simulink model "test_WaveletTraj"  (Simulink 10.1)
settings: Solver=FixedStepDiscrete  StartTime=0.0  StopTime=7  FixedStep=Ts  RelTol=1e-3
PreLoadFcn:
  | load param
undefined symbols (not defined in the file or in its folder): c_maxsz, DiscIntNeverNeededParam, Dphival_fi, f, interp_gain, interp_uplim, phival_fi, Ts, tval_fi, w
libraries: simulink x11, dspsigops x6, dspswit3 x3, simulink_extras x2, dspsrcs4 x1
settings Model: Creator=Carchesion  LastModifiedBy=upattacini  ParamWorkspaceSource=ReferencedWorkspace
settings SolverCC: ZeroCrossAlgorithm=Non-adaptive
settings DataIOCC: SignalLoggingSaveFormat=ModelDataLogs  SaveOutput=off  SignalLogging=off  SaveTime=off
settings OptimizationCC: DefaultParameterBehavior=Inlined  InlineInvariantSignals=on  ExpressionDepthLimit=2147483647  StateBitsets=on  DataBitsets=on  NoFixptDivByZeroProtection=on  EfficientFloat2IntCast=on  LifeSpan=1  SimCompilerOptimization=on  EfficientTunableParamExpr=on
settings DebuggingCC: SolverPrmCheckMsg=warning  ParameterPrecisionLossMsg=none  FcnCallInpInsideContextMsg=warning  StateNameClashWarn=warning
settings HardwareCC: ProdIntDivRoundTo=Zero  ProdEndianess=BigEndian  ProdWordSize=16  ProdHWDeviceType=Generic->Custom  TargetBitPerInt=16  TargetIntDivRoundTo=Zero  TargetEndianess=BigEndian  TargetWordSize=16  TargetHWDeviceType=Freescale->DSP563xx (16-bit mode)
settings SFSimCC: SimUseLocalCustomCode=on  SimParseCustomCode=off  MATLABDynamicMemAlloc=off  CustomCodeUndefinedFunction=FilterOut
settings RTWCC: Description=Real-Time Workshop Embedded Coder (no auto configuration)  SystemTargetFile=ert.tlc  GenCodeOnly=on  GenerateMakefile=off  TemplateMakefile=ert_default_tmf  GenerateReport=on  RTWUseLocalCustomCode=on  IncludeHyperlinkInReport=on  LaunchReport=on  PortableWordSizes=on  CreateSILPILBlock=SIL  GenerateTraceInfo=on  RTWCompilerOptimization=on
settings CodeAppCC: ForceParamTrailComments=on  IgnoreCustomStorageClasses=off  SimulinkDataObjDesc=on  CustomSymbolStrType=$R$N$M  CustomSymbolStrFcn=$N$M$F  CustomSymbolStrMacro=$N$M  InsertBlockDesc=on  InternalIdentifier=Classic
settings ERTTargetCC: GenerateSampleERTMain=on  IncludeMdlTerminateFcn=off  SuppressErrorStatus=on  PurelyIntegerCode=on  SupportNonFinite=off  SupportComplex=off  InlinedParameterPlacement=NonHierarchical  ERTCustomFileTemplate=example_file_process.tlc  GlobalDataDefinition=InSourceFile  GlobalDataReference=InSourceFile  ConvertIfToSwitch=off  SuppressUnreachableDefaultCases=off
settings ConfigComp: CovExternalEMLEnable=on

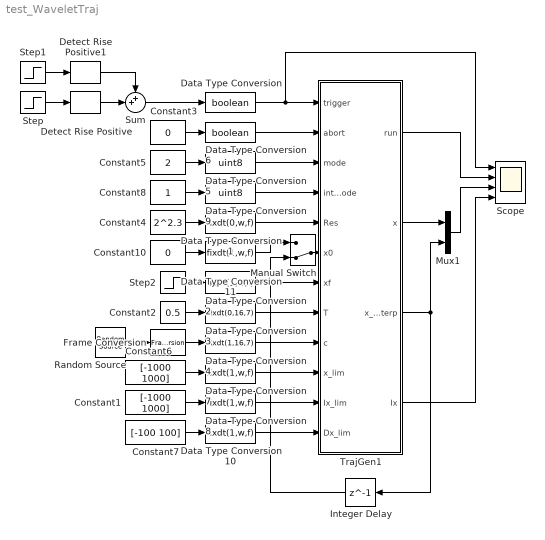
== system test_WaveletTraj ==
  Constant1 : Constant  Value=[-1000 1000]
  Constant10 : Constant  Value=0
  Constant2 : Constant  Value=0.5
  Constant3 : Constant  Value=0
  Constant4 : Constant  Value=2^2.3
  Constant5 : Constant  Value=2
  Constant6 : Constant  Value=[-1000 1000]
  Constant7 : Constant  Value=[-100 100]
  Constant8 : Constant
  Data Type Conversion : DataTypeConversion  OutDataTypeStr=boolean  RndMeth=Nearest  SaturateOnIntegerOverflow=on
  Data Type Conversion1 : DataTypeConversion  OutDataTypeStr=fixdt(0,w,f)  RndMeth=Nearest  SaturateOnIntegerOverflow=on
  Data Type Conversion{2,7..8,10..11} (5 alike) : DataTypeConversion  OutDataTypeStr=fixdt(1,w,f)  RndMeth=Nearest  SaturateOnIntegerOverflow=on
  Data Type Conversion3 : DataTypeConversion  OutDataTypeStr=fixdt(0,16,7)  RndMeth=Nearest  SaturateOnIntegerOverflow=on
  Data Type Conversion4 : DataTypeConversion  OutDataTypeStr=fixdt(1,16,7)  RndMeth=Nearest  SaturateOnIntegerOverflow=on
  Data Type Conversion5 : DataTypeConversion  OutDataTypeStr=uint8  RndMeth=Nearest  SaturateOnIntegerOverflow=on
  Data Type Conversion6 : DataTypeConversion  OutDataTypeStr=boolean  RndMeth=Nearest  SaturateOnIntegerOverflow=on
  Data Type Conversion9 : DataTypeConversion  OutDataTypeStr=uint8  RndMeth=Nearest  SaturateOnIntegerOverflow=on
  Detect Rise Positive : simulink/Logic and Bit Operations/Detect Rise Positive  vinit=0  OutDataTypeStr=uint8
  Detect Rise Positive1 : simulink/Logic and Bit Operations/Detect Rise Positive  vinit=0  OutDataTypeStr=uint8
  Frame Conversion : FrameConversion  OutFrame=Sample-based
  Integer Delay : Delay  DelayLength=1
  Manual Switch : ManualSwitch  CurrentSetting=0
  Mux1 : Mux  Inputs=2
  Random Source : dspsrcs4/Random Source  SrcType=Uniform  NormMethod=Ziggurat  CltLength=12  MinVal=-10  MaxVal=10  MeanVal=0  VarVal=1  RepMode=Not repeatable  rawSeed=1  IsInherit=off  SampMode=Discrete  SampTime=Ts/c_maxsz  SampFrame=c_maxsz  DataType=Double  OutComplex=Real  OutputFrames=on
  Scope : Scope  NumInputPorts=4
  Step : Step  SampleTime=Ts
  Step1 : Step  Time=2  SampleTime=Ts
  Step2 : Step  Time=1.5  Before=10  After=20  SampleTime=Ts
  Sum : Sum  Inputs=++|
  TrajGen1 : Subsystem  TreatAsAtomicUnit=on  RTWFcnName=WaveletTrajectory
      settings: RTWFcnNameOpts=User specified
  wires:
  Constant4/1 -> Data Type Conversion1/1
  Constant2/1 -> Data Type Conversion3/1
  Step/1 -> Detect Rise Positive/1
  Step1/1 -> Detect Rise Positive1/1
  Random Source/1 -> Frame Conversion/1
  Frame Conversion/1 -> Data Type Conversion4/1
  Data Type Conversion/1 -> Scope/1, TrajGen1/1(trigger)
  Sum/1 -> Data Type Conversion/1
  Mux1/1 -> Scope/3
  Data Type Conversion4/1 -> TrajGen1/9(c)
  Data Type Conversion3/1 -> TrajGen1/8(T)
  Data Type Conversion1/1 -> TrajGen1/5(Res)
  Step2/1 -> Data Type Conversion2/1
  Data Type Conversion2/1 -> TrajGen1/7(xf)
  Detect Rise Positive/1 -> Sum/2
  Detect Rise Positive1/1 -> Sum/1
  Data Type Conversion5/1 -> TrajGen1/3(mode)
  Data Type Conversion6/1 -> TrajGen1/2(abort)
  Constant5/1 -> Data Type Conversion5/1
  Data Type Conversion7/1 -> TrajGen1/10(x_lim)
  Data Type Conversion8/1 -> TrajGen1/11(Ix_lim)
  Constant6/1 -> Data Type Conversion7/1
  Constant1/1 -> Data Type Conversion8/1
  Constant3/1 -> Data Type Conversion6/1
  Constant8/1 -> Data Type Conversion9/1
  Data Type Conversion9/1 -> TrajGen1/4(int_mode)
  TrajGen1/1(run) -> Scope/2
  TrajGen1/2(x) -> Mux1/1
  TrajGen1/3(x_interp) -> Mux1/2, Integer Delay/1
  TrajGen1/4(Ix) -> Scope/4
  Data Type Conversion10/1 -> TrajGen1/12(Dx_lim)
  Constant7/1 -> Data Type Conversion10/1
  Manual Switch/1 -> TrajGen1/6(x0)
  Integer Delay/1 -> Manual Switch/2
  Constant10/1 -> Data Type Conversion11/1
  Data Type Conversion11/1 -> Manual Switch/1

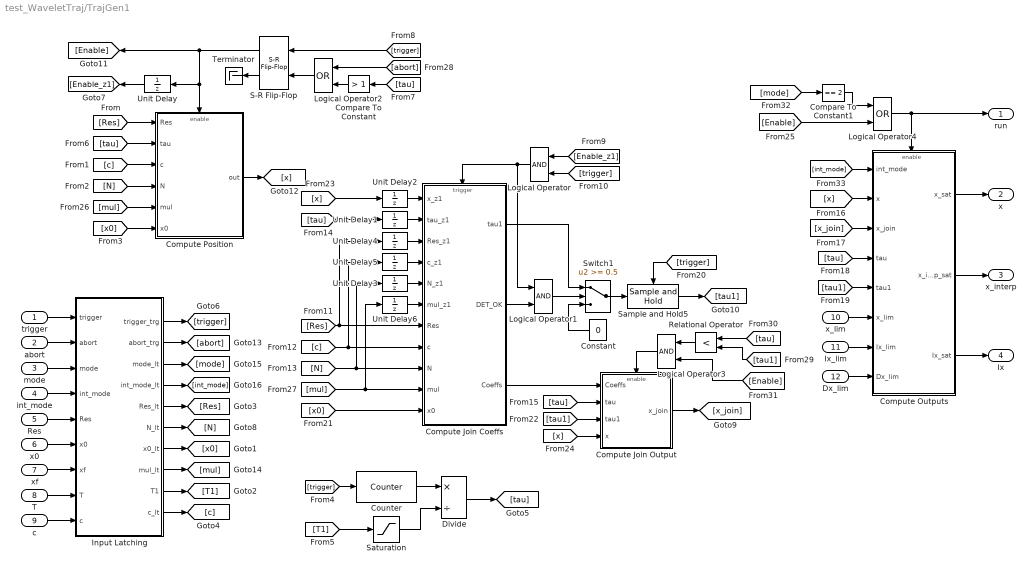
== system test_WaveletTraj/TrajGen1 ==
  trigger : Inport  PortDimensions=1
  abort : Inport  Port=2  PortDimensions=1
  mode : Inport  Port=3  PortDimensions=1
  int_mode : Inport  Port=4  PortDimensions=1
  Res : Inport  Port=5  PortDimensions=1
  x0 : Inport  Port=6  PortDimensions=1
  xf : Inport  Port=7  PortDimensions=1
  T : Inport  Port=8  PortDimensions=1
  c : Inport  Port=9  PortDimensions=c_maxsz
  x_lim : Inport  Port=10  PortDimensions=2
  Ix_lim : Inport  Port=11  PortDimensions=2
  Dx_lim : Inport  Port=12  PortDimensions=2
  Compare To Constant : simulink/Logic and Bit Operations/Compare To Constant  relop=>  const=1  OutDataTypeStr=boolean  ZeroCross=off
  Compare To Constant1 : simulink/Logic and Bit Operations/Compare To Constant  relop===  const=2  OutDataTypeStr=boolean  ZeroCross=off
  Compute Join Coeffs : Subsystem  RTWFcnName=Trajectory_ComputeJoinCoeffs
      settings: RTWFcnNameOpts=User specified
  Compute Join Output : Subsystem  TreatAsAtomicUnit=on  RTWFcnName=Trajectory_ComputeJoinOutput
      settings: RTWFcnNameOpts=User specified
  Compute Outputs : Subsystem  TreatAsAtomicUnit=on  RTWFcnName=Trajectory_ComputeOutputs
      settings: RTWFcnNameOpts=User specified
  Compute Position : Subsystem  TreatAsAtomicUnit=on  RTWFcnName=Trajectory_ComputePosition
      settings: RTWFcnNameOpts=User specified
  Constant : Constant  Value=0  OutDataTypeStr=fixdt(1,w,f)
  Counter : dspswit3/Counter  Direction=Up  CountEvent=Free running  CounterSize=32 bits  MaxCount=255  InitialCount=0  Output=Count  HitValue=32  ResetInput=on  SamplesPerFrame=1  Ts=-1  CntDtype=uint32  HitDtype=Logical
  Divide : Product  Inputs=*/  OutDataTypeStr=fixdt(1,w,f)  RndMeth=Nearest  SaturateOnIntegerOverflow=on
  Input Latching : Subsystem  TreatAsAtomicUnit=on  RTWFcnName=Trajectory_InputLatching
      settings: RTWFcnNameOpts=User specified
  Logical Operator : Logic  IconShape=distinctive  AllPortsSameDT=off  OutDataTypeStr=boolean
  Logical Operator1 : Logic  IconShape=distinctive  AllPortsSameDT=off  OutDataTypeStr=boolean
  Logical Operator2 : Logic  Operator=OR  IconShape=distinctive  AllPortsSameDT=off  OutDataTypeStr=boolean
  Logical Operator3 : Logic  IconShape=distinctive  AllPortsSameDT=off  OutDataTypeStr=boolean
  Logical Operator4 : Logic  Operator=OR  IconShape=distinctive  AllPortsSameDT=off  OutDataTypeStr=boolean
  Relational Operator : RelationalOperator  Operator=<  OutDataTypeStr=boolean  RndMeth=Nearest
  S-R Flip-Flop : simulink_extras/Flip Flops/S-R Flip-Flop  initial_condition=0
  Sample and Hold5 : dspsigops/Sample and Hold  trig=Rising edge  initCond=0  latchinput=off
  Saturation : Saturate  UpperLimit=intmax('uint32')  LowerLimit=1  OutDataTypeStr=uint32  RndMeth=Nearest
  Switch1 : Switch  Threshold=0.5  OutDataTypeStr=fixdt(0,w,f)  RndMeth=Nearest  SaturateOnIntegerOverflow=on
  Terminator : Terminator
  Unit Delay{,1..6} (7 alike) : UnitDelay  SampleTime=-1
  run : Outport  PortDimensions=1
  x : Outport  Port=2  PortDimensions=1
  x_interp : Outport  Port=3  PortDimensions=1
  Ix : Outport  Port=4  PortDimensions=1
  wires:
  Unit Delay4/1 -> Compute Join Coeffs/3(Res_z1)
  [x] -> Compute Join Output/4(x)
  [tau1] -> Compute Join Output/3(tau1)
  Compute Join Output/1(x_join) -> [x_join]
  Unit Delay2/1 -> Compute Join Coeffs/1(x_z1)
  Unit Delay1/1 -> Compute Join Coeffs/2(tau_z1)
  [x0] -> Compute Position/6(x0)
  [x] -> Unit Delay2/1
  [tau] -> Unit Delay1/1
  Logical Operator1/1 -> Switch1/2
  Compute Join Coeffs/2(DET_OK) -> Logical Operator1/2
  [x0] -> Compute Join Coeffs/11(x0)
  [tau] -> Compute Join Output/2(tau)
  Compute Join Coeffs/3(Coeffs) -> Compute Join Output/1(Coeffs)
  [trigger] -> Sample and Hold5/Trigger
  Sample and Hold5/1 -> [tau1]
  Constant/1 -> Switch1/3
  Compute Join Coeffs/1(tau1) -> Switch1/1
  Switch1/1 -> Sample and Hold5/1
  Logical Operator/1 -> Logical Operator1/1, Compute Join Coeffs/Trigger
  [N] -> Compute Join Coeffs/9(N), Unit Delay3/1
  [c] -> Compute Join Coeffs/8(c), Unit Delay5/1
  [Res] -> Unit Delay4/1, Compute Join Coeffs/7(Res)
  Compute Position/1(out) -> [x]
  [trigger] -> Logical Operator/2
  [Enable_z1] -> Logical Operator/1
  [trigger] -> Counter/1
  Counter/1 -> Divide/1
  S-R Flip-Flop/1 -> Compute Position/Enable, Unit Delay/1, [Enable]
  S-R Flip-Flop/2 -> Terminator/1
  [tau] -> Compare To Constant/1
  [trigger] -> S-R Flip-Flop/1
  Saturation/1 -> Divide/2
  [tau] -> Compute Position/2(tau)
  Divide/1 -> [tau]
  [T1] -> Saturation/1
  [N] -> Compute Position/4(N)
  [c] -> Compute Position/3(c)
  [Res] -> Compute Position/1(Res)
  Unit Delay5/1 -> Compute Join Coeffs/4(c_z1)
  Unit Delay3/1 -> Compute Join Coeffs/5(N_z1)
  Unit Delay/1 -> [Enable_z1]
  trigger/1 -> Input Latching/1(trigger)
  mode/1 -> Input Latching/3(mode)
  Res/1 -> Input Latching/5(Res)
  x0/1 -> Input Latching/6(x0)
  T/1 -> Input Latching/8(T)
  c/1 -> Input Latching/9(c)
  xf/1 -> Input Latching/7(xf)
  Input Latching/1(trigger_trg) -> [trigger]
  Input Latching/5(Res_lt) -> [Res]
  Input Latching/6(N_lt) -> [N]
  Input Latching/7(x0_lt) -> [x0]
  Input Latching/9(T1) -> [T1]
  Input Latching/10(c_lt) -> [c]
  Input Latching/8(mul_lt) -> [mul]
  [mul] -> Compute Position/5(mul)
  [mul] -> Compute Join Coeffs/10(mul), Unit Delay6/1
  Unit Delay6/1 -> Compute Join Coeffs/6(mul_z1)
  abort/1 -> Input Latching/2(abort)
  Input Latching/2(abort_trg) -> [abort]
  Logical Operator2/1 -> S-R Flip-Flop/2
  [abort] -> Logical Operator2/1
  x_lim/1 -> Compute Outputs/6(x_lim)
  Ix_lim/1 -> Compute Outputs/7(Ix_lim)
  [tau1] -> Compute Outputs/5(tau1)
  [tau] -> Compute Outputs/4(tau)
  [x_join] -> Compute Outputs/3(x_join)
  [x] -> Compute Outputs/2(x)
  Compute Outputs/1(x_sat) -> x/1
  Compute Outputs/2(x_interp_sat) -> x_interp/1
  Compute Outputs/3(Ix_sat) -> Ix/1
  [tau] -> Relational Operator/1
  [tau1] -> Relational Operator/2
  Relational Operator/1 -> Logical Operator3/1
  Logical Operator3/1 -> Compute Join Output/Enable
  [Enable] -> Logical Operator3/2
  Dx_lim/1 -> Compute Outputs/8(Dx_lim)
  int_mode/1 -> Input Latching/4(int_mode)
  Input Latching/3(mode_lt) -> [mode]
  Input Latching/4(int_mode_lt) -> [int_mode]
  [int_mode] -> Compute Outputs/1(int_mode)
  [mode] -> Compare To Constant1/1
  Compare To Constant/1 -> Logical Operator2/2
  [Enable] -> Logical Operator4/2
  Logical Operator4/1 -> Compute Outputs/Enable, run/1
  Compare To Constant1/1 -> Logical Operator4/1

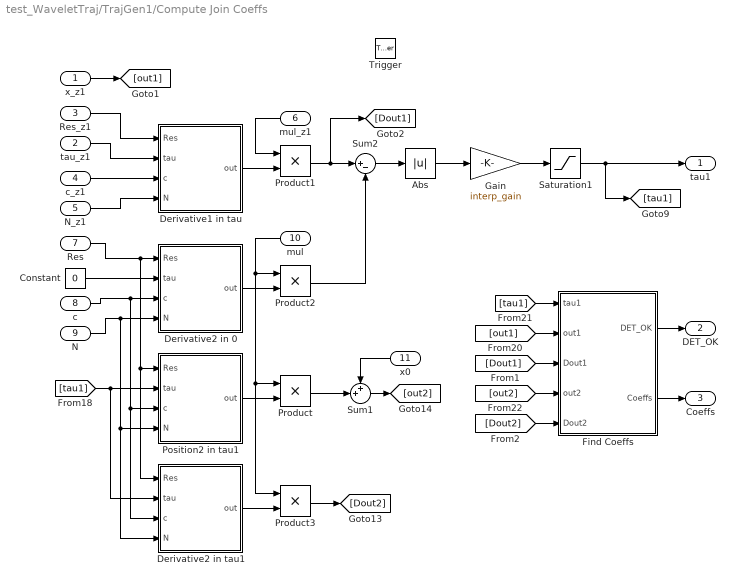
== system test_WaveletTraj/TrajGen1/Compute Join Coeffs ==
  x_z1 : Inport
  tau_z1 : Inport  Port=2
  Res_z1 : Inport  Port=3
  c_z1 : Inport  Port=4
  N_z1 : Inport  Port=5
  mul_z1 : Inport  Port=6
  Res : Inport  Port=7
  c : Inport  Port=8
  N : Inport  Port=9
  mul : Inport  Port=10
  x0 : Inport  Port=11
  Trigger : TriggerPort  VariantControl=(inherit)  StatesWhenEnabling=reset
  Abs : Abs  RndMeth=Nearest  SaturateOnIntegerOverflow=on
  Constant : Constant  Value=0  OutDataTypeStr=fixdt(1,w,f)
  Derivative1 in tau : Subsystem  TreatAsAtomicUnit=on  RTWFcnName=Trajectory_Derivative
      settings: RTWFcnNameOpts=User specified
  Derivative2 in 0 : Subsystem  TreatAsAtomicUnit=on  RTWFcnName=Trajectory_Derivative
      settings: RTWFcnNameOpts=User specified
  Derivative2 in tau1 : Subsystem  TreatAsAtomicUnit=on  RTWFcnName=Trajectory_Derivative
      settings: RTWFcnNameOpts=User specified
  Find Coeffs : Subsystem  TreatAsAtomicUnit=on  RTWFcnName=Trajectory_FindCoeffs
      settings: RTWFcnNameOpts=User specified
  Gain : Gain  Gain=interp_gain  ParamDataTypeStr=fixdt(1,w,f)  RndMeth=Nearest  SaturateOnIntegerOverflow=on  OutDataTypeStr=Inherit: Same as input
  Position2 in tau1 : Subsystem  TreatAsAtomicUnit=on  RTWFcnName=Trajectory_Position
      settings: RTWFcnNameOpts=User specified
  Product{,1..3} (4 alike) : Product  OutDataTypeStr=fixdt(1,w,f)  RndMeth=Nearest  SaturateOnIntegerOverflow=on
  Saturation1 : Saturate  UpperLimit=interp_uplim  LowerLimit=0  OutDataTypeStr=fixdt(1,w,f)  RndMeth=Nearest
  Sum1 : Sum  Inputs=++|  OutDataTypeStr=fixdt(1,w,f)  RndMeth=Nearest  SaturateOnIntegerOverflow=on
  Sum2 : Sum  Inputs=|+-  OutDataTypeStr=fixdt(1,w,f)  RndMeth=Nearest  SaturateOnIntegerOverflow=on
  tau1 : Outport
  DET_OK : Outport  Port=2
  Coeffs : Outport  Port=3
  wires:
  N_z1/1 -> Derivative1 in tau/4(N)
  Res_z1/1 -> Derivative1 in tau/1(Res)
  Find Coeffs/1(DET_OK) -> DET_OK/1
  tau_z1/1 -> Derivative1 in tau/2(tau)
  c_z1/1 -> Derivative1 in tau/3(c)
  x0/1 -> Sum1/1
  Sum1/1 -> [out2]
  Saturation1/1 -> [tau1], tau1/1
  Find Coeffs/2(Coeffs) -> Coeffs/1
  [Dout2] -> Find Coeffs/5(Dout2)
  [out2] -> Find Coeffs/4(out2)
  [Dout1] -> Find Coeffs/3(Dout1)
  [out1] -> Find Coeffs/2(out1)
  [tau1] -> Find Coeffs/1(tau1)
  x_z1/1 -> [out1]
  [tau1] -> Derivative2 in tau1/2(tau), Position2 in tau1/2(tau)
  Gain/1 -> Saturation1/1
  Abs/1 -> Gain/1
  Sum2/1 -> Abs/1
  N/1 -> Derivative2 in 0/4(N), Derivative2 in tau1/4(N), Position2 in tau1/4(N)
  c/1 -> Derivative2 in 0/3(c), Derivative2 in tau1/3(c), Position2 in tau1/3(c)
  Constant/1 -> Derivative2 in 0/2(tau)
  Res/1 -> Derivative2 in 0/1(Res), Derivative2 in tau1/1(Res), Position2 in tau1/1(Res)
  Product/1 -> Sum1/2
  Derivative1 in tau/1(out) -> Product1/2
  Product1/1 -> Sum2/1, [Dout1]
  mul_z1/1 -> Product1/1
  Derivative2 in 0/1(out) -> Product2/2
  Product2/1 -> Sum2/2
  Derivative2 in tau1/1(out) -> Product3/2
  Product3/1 -> [Dout2]
  Position2 in tau1/1(out) -> Product/2
  mul/1 -> Product2/1, Product/1, Product3/1

== system test_WaveletTraj/TrajGen1/Compute Join Output ==
  Coeffs : Inport
  tau : Inport  Port=2
  tau1 : Inport  Port=3
  x : Inport  Port=4
  Enable : EnablePort
  CalcPoly : Subsystem
  CalcRho : Subsystem
  Product : Product  OutDataTypeStr=fixdt(1,w,f)  RndMeth=Nearest  SaturateOnIntegerOverflow=on
  Product1 : Product  OutDataTypeStr=fixdt(1,w,f)  RndMeth=Nearest  SaturateOnIntegerOverflow=on
  Sum2 : Sum  Inputs=|++  OutDataTypeStr=fixdt(1,w,f)  RndMeth=Nearest  SaturateOnIntegerOverflow=on
  x_join : Outport
  wires:
  x/1 -> Product1/2
  CalcRho/2(Rho2) -> Product1/1
  Sum2/1 -> x_join/1
  Product1/1 -> Sum2/2
  Product/1 -> Sum2/1
  CalcRho/1(Rho1) -> Product/2
  CalcPoly/1(out_poly3) -> Product/1
  tau1/1 -> CalcRho/2(tau1)
  Coeffs/1 -> CalcPoly/2(Coeffs)
  tau/1 -> CalcRho/1(tau), CalcPoly/1(tau)

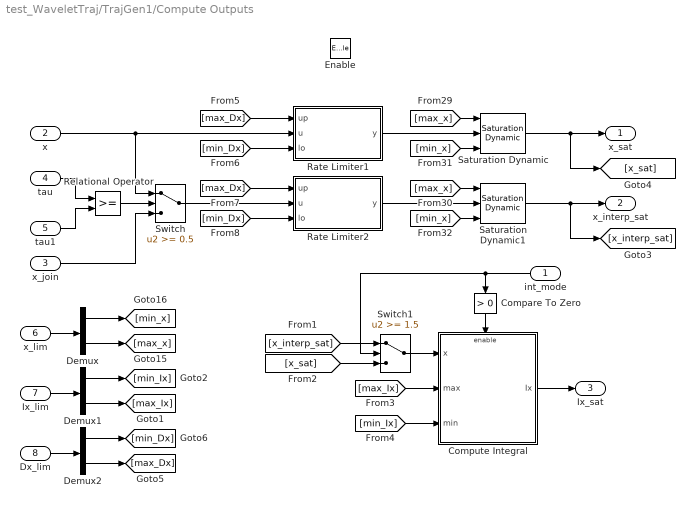
== system test_WaveletTraj/TrajGen1/Compute Outputs ==
  int_mode : Inport
  x : Inport  Port=2
  x_join : Inport  Port=3
  tau : Inport  Port=4
  tau1 : Inport  Port=5
  x_lim : Inport  Port=6
  Ix_lim : Inport  Port=7
  Dx_lim : Inport  Port=8
  Enable : EnablePort
  Compare To Zero : simulink/Logic and Bit Operations/Compare To Zero  relop=>  OutDataTypeStr=boolean  ZeroCross=off
  Compute Integral : Subsystem  TreatAsAtomicUnit=on  RTWFcnName=Trajectory_ComputeIntegral
      settings: RTWFcnNameOpts=User specified
  Demux : Demux  Outputs=2
  Demux1 : Demux  Outputs=2
  Demux2 : Demux  Outputs=2
  Rate Limiter1 : Subsystem  TreatAsAtomicUnit=on  RTWFcnName=Trajectory_RateLimiter
      settings: RTWFcnNameOpts=User specified
      mask Display:
      | disp('Rate\nLimiter');
      | port_label('input',1,'up');
      | port_label('input',2,'u');
      | port_label('input',3,'lo');
      | port_label('output',1,'y');
  Rate Limiter2 : Subsystem  TreatAsAtomicUnit=on  RTWFcnName=Trajectory_RateLimiter
      settings: RTWFcnNameOpts=User specified
      mask Display:
      | disp('Rate\nLimiter');
      | port_label('input',1,'up');
      | port_label('input',2,'u');
      | port_label('input',3,'lo');
      | port_label('output',1,'y');
  Relational Operator : RelationalOperator  OutDataTypeStr=boolean  RndMeth=Nearest
  Saturation Dynamic : simulink/Discontinuities/Saturation Dynamic  OutMin=[]  OutMax=[]  OutDataTypeStr=fixdt(1,w,f)  OutputDataTypeScalingMode=Specify via dialog  OutDataType=fixdt(1,w,f)  OutScaling=[]  RndMeth=Nearest  DoSatur=on
  Saturation Dynamic1 : simulink/Discontinuities/Saturation Dynamic  OutMin=[]  OutMax=[]  OutDataTypeStr=fixdt(1,w,f)  OutputDataTypeScalingMode=Specify via dialog  OutDataType=fixdt(1,w,f)  OutScaling=[]  RndMeth=Nearest  DoSatur=on
  Switch : Switch  Threshold=0.5  OutDataTypeStr=fixdt(1,w,f)  RndMeth=Nearest  SaturateOnIntegerOverflow=on
  Switch1 : Switch  Threshold=1.5  OutDataTypeStr=fixdt(1,w,f)  RndMeth=Nearest  SaturateOnIntegerOverflow=on
  x_sat : Outport
  x_interp_sat : Outport  Port=2
  Ix_sat : Outport  Port=3
  wires:
  x/1 -> Switch/1, Rate Limiter1/2(u)
  [min_x] -> Saturation Dynamic1/3
  [min_x] -> Saturation Dynamic/3
  [max_x] -> Saturation Dynamic1/1
  [max_x] -> Saturation Dynamic/1
  Relational Operator/1 -> Switch/2
  Saturation Dynamic/1 -> x_sat/1, [x_sat]
  tau/1 -> Relational Operator/1
  Saturation Dynamic1/1 -> x_interp_sat/1, [x_interp_sat]
  tau1/1 -> Relational Operator/2
  x_join/1 -> Switch/3
  Demux/1 -> [min_x]
  Demux/2 -> [max_x]
  Demux1/1 -> [min_Ix]
  Demux1/2 -> [max_Ix]
  [max_Ix] -> Compute Integral/2(max)
  [min_Ix] -> Compute Integral/3(min)
  Compute Integral/1(Ix) -> Ix_sat/1
  x_lim/1 -> Demux/1
  Ix_lim/1 -> Demux1/1
  [x_interp_sat] -> Switch1/1
  [x_sat] -> Switch1/3
  Switch1/1 -> Compute Integral/1(x)
  int_mode/1 -> Compare To Zero/1, Switch1/2
  Compare To Zero/1 -> Compute Integral/Enable
  Demux2/1 -> [min_Dx]
  Demux2/2 -> [max_Dx]
  Dx_lim/1 -> Demux2/1
  Rate Limiter1/1(y) -> Saturation Dynamic/2
  Rate Limiter2/1(y) -> Saturation Dynamic1/2
  Switch/1 -> Rate Limiter2/2(u)
  [max_Dx] -> Rate Limiter1/1(up)
  [min_Dx] -> Rate Limiter1/3(lo)
  [min_Dx] -> Rate Limiter2/3(lo)
  [max_Dx] -> Rate Limiter2/1(up)

== system test_WaveletTraj/TrajGen1/Compute Position ==
  Res : Inport  PortDimensions=1
  tau : Inport  Port=2  PortDimensions=1
  c : Inport  Port=3  PortDimensions=c_maxsz
  N : Inport  Port=4  PortDimensions=1
  mul : Inport  Port=5  PortDimensions=1
  x0 : Inport  Port=6  PortDimensions=1
  Enable : EnablePort
  Position : Subsystem  TreatAsAtomicUnit=on  RTWFcnName=Trajectory_Position
      settings: RTWFcnNameOpts=User specified
  Product : Product  OutDataTypeStr=fixdt(1,w,f)  RndMeth=Nearest  SaturateOnIntegerOverflow=on
  Sum1 : Sum  Inputs=|++  OutDataTypeStr=fixdt(1,w,f)  RndMeth=Nearest  SaturateOnIntegerOverflow=on
  out : Outport  PortDimensions=1
  wires:
  x0/1 -> Sum1/2
  Sum1/1 -> out/1
  N/1 -> Position/4(N)
  c/1 -> Position/3(c)
  tau/1 -> Position/2(tau)
  Res/1 -> Position/1(Res)
  Position/1(out) -> Product/1
  Product/1 -> Sum1/1
  mul/1 -> Product/2

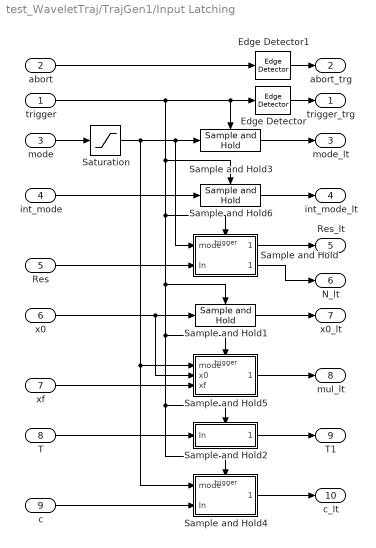
== system test_WaveletTraj/TrajGen1/Input Latching ==
  trigger : Inport
  abort : Inport  Port=2
  mode : Inport  Port=3
  int_mode : Inport  Port=4
  Res : Inport  Port=5
  x0 : Inport  Port=6
  xf : Inport  Port=7
  T : Inport  Port=8
  c : Inport  Port=9
  Edge Detector : dspswit3/Edge Detector  InputProcessing=Columns as channels (frame based)
      settings: SourceProductBaseCode=DS
  Edge Detector1 : dspswit3/Edge Detector  InputProcessing=Columns as channels (frame based)
      settings: SourceProductBaseCode=DS
  Sample and Hold : Subsystem  TreatAsAtomicUnit=on  mask(Sample and Hold){trig=Rising edge, initCond=0, latchinput=off}
      mask prompts: trig "Trigger type:"; initCond "Initial condition:"; latchinput "Latch (buffer) input"
      mask help: Sample and hold the input signal. If Latch (buffer) input is selected, then this block produces the value of the input from the previous time step.
      mask init:
      | switch trig
      | case 1, s='rising';
      | case 2, s='falling';
      | case 3, s='either';
      | end
      | set_param([gcb '/Trigger'],'triggertype',s);
      | if (latchinput == 1)
      | 	set_param([gcb '/In'],'latchinput','on');
      | 	set_param([gcb '/mode'],'latchinput','on');
      | else
      | 	set_param([gcb '/In'],'latchinput','off');
      | 	set_param([gcb '/mode'],'latchinput','off');
      | end
      mask Help: eval('blocksethelp');
      mask TypeOptions trig: Rising edge | Falling edge | Either edge
      mask Display: disp('S/H')
  Sample and Hold1 : dspsigops/Sample and Hold  trig=Rising edge  initCond=0  latchinput=off
  Sample and Hold2 : Subsystem  TreatAsAtomicUnit=on  mask(Sample and Hold){trig=Rising edge, initCond=0, latchinput=off}
      mask prompts: trig "Trigger type:"; initCond "Initial condition:"; latchinput "Latch (buffer) input"
      mask help: Sample and hold the input signal. If Latch (buffer) input is selected, then this block produces the value of the input from the previous time step.
      mask init:
      | switch trig
      | case 1, s='rising';
      | case 2, s='falling';
      | case 3, s='either';
      | end
      | set_param([gcb '/Trigger'],'triggertype',s);
      | if (latchinput == 1)
      | 	set_param([gcb '/In'],'latchinput','on');
      | else
      | 	set_param([gcb '/In'],'latchinput','off');
      | end
      mask Help: eval('blocksethelp');
      mask TypeOptions trig: Rising edge | Falling edge | Either edge
      mask Display: disp('S/H')
  Sample and Hold3 : dspsigops/Sample and Hold  trig=Rising edge  initCond=0  latchinput=off
  Sample and Hold4 : Subsystem  TreatAsAtomicUnit=on  mask(Sample and Hold){trig=Rising edge, initCond=0, latchinput=off}
      mask prompts: trig "Trigger type:"; initCond "Initial condition:"; latchinput "Latch (buffer) input"
      mask help: Sample and hold the input signal. If Latch (buffer) input is selected, then this block produces the value of the input from the previous time step.
      mask init: same as test_WaveletTraj/TrajGen1/Input Latching/Sample and Hold
      mask Help: eval('blocksethelp');
      mask TypeOptions trig: Rising edge | Falling edge | Either edge
      mask Display: disp('S/H')
  Sample and Hold5 : Subsystem  TreatAsAtomicUnit=on  mask(Sample and Hold){trig=Rising edge, initCond=0, latchinput=off}
      mask prompts: trig "Trigger type:"; initCond "Initial condition:"; latchinput "Latch (buffer) input"
      mask help: Sample and hold the input signal. If Latch (buffer) input is selected, then this block produces the value of the input from the previous time step.
      mask init:
      | switch trig
      | case 1, s='rising';
      | case 2, s='falling';
      | case 3, s='either';
      | end
      | set_param([gcb '/Trigger'],'triggertype',s);
      | if (latchinput == 1)
      | 	set_param([gcb '/mode'],'latchinput','on');
      | 	set_param([gcb '/x0'],'latchinput','on');
      | 	set_param([gcb '/xf'],'latchinput','on');
      | else
      | 	set_param([gcb '/mode'],'latchinput','off');
      | 	set_param([gcb '/x0'],'latchinput','off');
      | 	set_param([gcb '/xf'],'latchinput','off');
      | end
      mask Help: eval('blocksethelp');
      mask TypeOptions trig: Rising edge | Falling edge | Either edge
      mask Display: disp('S/H')
  Sample and Hold6 : dspsigops/Sample and Hold  trig=Rising edge  initCond=0  latchinput=off
  Saturation : Saturate  UpperLimit=2  LowerLimit=0  OutDataTypeStr=uint8  RndMeth=Nearest
  trigger_trg : Outport
  abort_trg : Outport  Port=2
  mode_lt : Outport  Port=3
  int_mode_lt : Outport  Port=4
  Res_lt : Outport  Port=5
  N_lt : Outport  Port=6
  x0_lt : Outport  Port=7
  mul_lt : Outport  Port=8
  T1 : Outport  Port=9
  c_lt : Outport  Port=10
  wires:
  Sample and Hold4/1(" ") -> c_lt/1
  Sample and Hold2/1(" ") -> T1/1
  T/1 -> Sample and Hold2/1(In)
  Sample and Hold1/1 -> x0_lt/1
  x0/1 -> Sample and Hold1/1, Sample and Hold5/2(x0)
  Sample and Hold/2(" 1") -> N_lt/1
  Res/1 -> Sample and Hold/2(In)
  Sample and Hold/1(" ") -> Res_lt/1
  Edge Detector/1 -> trigger_trg/1
  trigger/1 -> Edge Detector/1, Sample and Hold3/Trigger, Sample and Hold1/Trigger, Sample and Hold5/Trigger, Sample and Hold2/Trigger, Sample and Hold4/Trigger, Sample and Hold/Trigger, Sample and Hold6/Trigger
  mode/1 -> Saturation/1
  xf/1 -> Sample and Hold5/3(xf)
  Sample and Hold5/1(" ") -> mul_lt/1
  c/1 -> Sample and Hold4/2(In)
  abort/1 -> Edge Detector1/1
  Edge Detector1/1 -> abort_trg/1
  Sample and Hold3/1 -> mode_lt/1
  Sample and Hold6/1 -> int_mode_lt/1
  int_mode/1 -> Sample and Hold6/1
  Saturation/1 -> Sample and Hold4/1(mode), Sample and Hold5/1(mode), Sample and Hold/1(mode), Sample and Hold3/1

== system test_WaveletTraj/TrajGen1/Compute Join Coeffs/Derivative1 in tau ==
  Res : Inport
  tau : Inport  Port=2
  c : Inport  Port=3
  N : Inport  Port=4
  Derivative : Subsystem  RTWFcnName=Trajectory_Derivative
  out : Outport
  wires:
  N/1 -> Derivative/4(N)
  c/1 -> Derivative/3(c)
  Derivative/1(Dout) -> out/1
  tau/1 -> Derivative/2(tau)
  Res/1 -> Derivative/1(Res)

== system test_WaveletTraj/TrajGen1/Compute Join Coeffs/Derivative2 in 0 ==
  Res : Inport
  tau : Inport  Port=2
  c : Inport  Port=3
  N : Inport  Port=4
  Derivative : Subsystem  RTWFcnName=Trajectory_Derivative
  out : Outport
  wires:
  Res/1 -> Derivative/1(Res)
  tau/1 -> Derivative/2(tau)
  Derivative/1(Dout) -> out/1
  c/1 -> Derivative/3(c)
  N/1 -> Derivative/4(N)

== system test_WaveletTraj/TrajGen1/Compute Join Coeffs/Derivative2 in tau1 ==
  Res : Inport
  tau : Inport  Port=2
  c : Inport  Port=3
  N : Inport  Port=4
  Derivative : Subsystem  RTWFcnName=Trajectory_Derivative
  out : Outport
  wires:
  N/1 -> Derivative/4(N)
  c/1 -> Derivative/3(c)
  Derivative/1(Dout) -> out/1
  tau/1 -> Derivative/2(tau)
  Res/1 -> Derivative/1(Res)

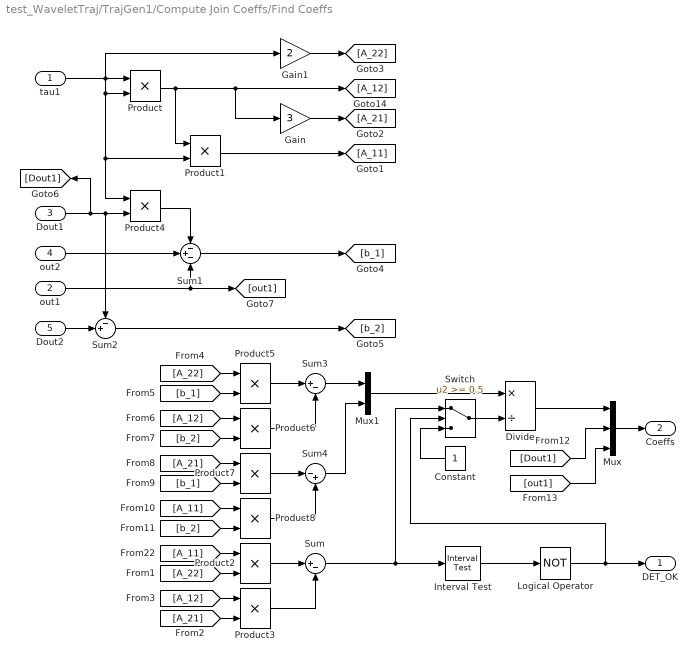
== system test_WaveletTraj/TrajGen1/Compute Join Coeffs/Find Coeffs ==
  tau1 : Inport
  out1 : Inport  Port=2
  Dout1 : Inport  Port=3
  out2 : Inport  Port=4
  Dout2 : Inport  Port=5
  Constant : Constant  OutDataTypeStr=fixdt(1,w,f)
  Divide : Product  Inputs=*/  OutDataTypeStr=fixdt(1,w,f)  RndMeth=Nearest  SaturateOnIntegerOverflow=on
  Gain : Gain  Gain=3  RndMeth=Nearest  SaturateOnIntegerOverflow=on  OutDataTypeStr=Inherit: Same as input  ParamDataTypeStr=Inherit: Same as input
  Gain1 : Gain  Gain=2  RndMeth=Nearest  SaturateOnIntegerOverflow=on  OutDataTypeStr=Inherit: Same as input  ParamDataTypeStr=Inherit: Same as input
  Interval Test : simulink/Logic and Bit Operations/Interval Test  IntervalClosedRight=on  uplimit=2^-f  IntervalClosedLeft=on  lowlimit=-2^-f  OutDataTypeStr=boolean
  Logical Operator : Logic  Operator=NOT  IconShape=distinctive  AllPortsSameDT=off  OutDataTypeStr=boolean
  Mux : Mux  Inputs=3
  Mux1 : Mux  Inputs=2
  Product{,1..8} (9 alike) : Product  OutDataTypeStr=fixdt(1,w,f)  RndMeth=Nearest  SaturateOnIntegerOverflow=on
  Sum : Sum  Inputs=|+-  OutDataTypeStr=fixdt(1,w,f)  RndMeth=Nearest  SaturateOnIntegerOverflow=on
  Sum1 : Sum  Inputs=-+-  OutDataTypeStr=fixdt(1,w,f)  RndMeth=Nearest  SaturateOnIntegerOverflow=on
  Sum2 : Sum  Inputs=-+|  OutDataTypeStr=fixdt(1,w,f)  RndMeth=Nearest  SaturateOnIntegerOverflow=on
  Sum3 : Sum  Inputs=|+-  OutDataTypeStr=fixdt(1,w,f)  RndMeth=Nearest  SaturateOnIntegerOverflow=on
  Sum4 : Sum  Inputs=|-+  OutDataTypeStr=fixdt(1,w,f)  RndMeth=Nearest  SaturateOnIntegerOverflow=on
  Switch : Switch  Threshold=0.5  OutDataTypeStr=fixdt(1,w,f)  RndMeth=Nearest  SaturateOnIntegerOverflow=on
  DET_OK : Outport
  Coeffs : Outport  Port=2
  wires:
  Constant/1 -> Switch/3
  Switch/1 -> Divide/2
  Logical Operator/1 -> Switch/2, DET_OK/1
  Interval Test/1 -> Logical Operator/1
  Mux/1 -> Coeffs/1
  [out1] -> Mux/3
  [Dout1] -> Mux/2
  Divide/1 -> Mux/1
  Sum/1 -> Switch/1, Interval Test/1
  Mux1/1 -> Divide/1
  Sum4/1 -> Mux1/2
  Sum3/1 -> Mux1/1
  Product8/1 -> Sum4/2
  Product7/1 -> Sum4/1
  [b_2] -> Product8/2
  [A_11] -> Product8/1
  [b_1] -> Product7/2
  [A_21] -> Product7/1
  Product6/1 -> Sum3/2
  Product5/1 -> Sum3/1
  [b_2] -> Product6/2
  [A_12] -> Product6/1
  [b_1] -> Product5/2
  [A_22] -> Product5/1
  Sum2/1 -> [b_2]
  Sum1/1 -> [b_1]
  Dout2/1 -> Sum2/2
  Product4/1 -> Sum1/1
  out1/1 -> [out1], Sum1/3
  out2/1 -> Sum1/2
  Dout1/1 -> [Dout1], Sum2/1, Product4/2
  Product3/1 -> Sum/2
  Product2/1 -> Sum/1
  [A_21] -> Product3/2
  [A_12] -> Product3/1
  [A_22] -> Product2/2
  [A_11] -> Product2/1
  Gain1/1 -> [A_22]
  Gain/1 -> [A_21]
  Product1/1 -> [A_11]
  Product/1 -> Gain/1, [A_12], Product1/1
  tau1/1 -> Gain1/1, Product4/1, Product1/2, Product/2, Product/1

== system test_WaveletTraj/TrajGen1/Compute Join Coeffs/Position2 in tau1 ==
  Res : Inport
  tau : Inport  Port=2
  c : Inport  Port=3
  N : Inport  Port=4
  Position : Subsystem  RTWFcnName=Trajectory_Position
  out : Outport
  wires:
  Res/1 -> Position/1(Res)
  tau/1 -> Position/2(tau)
  Position/1(out) -> out/1
  c/1 -> Position/3(c)
  N/1 -> Position/4(N)

== system test_WaveletTraj/TrajGen1/Compute Join Output/CalcPoly ==
  tau : Inport
  Coeffs : Inport  Port=2
  Add : Sum  Inputs=4  OutDataTypeStr=fixdt(1,w,f)  RndMeth=Nearest  SaturateOnIntegerOverflow=on
  Demux : Demux
  Product{,1..4} (5 alike) : Product  OutDataTypeStr=fixdt(1,w,f)  RndMeth=Nearest  SaturateOnIntegerOverflow=on
  out_poly3 : Outport
  wires:
  Coeffs/1 -> Demux/1
  Add/1 -> out_poly3/1
  Demux/4 -> Add/4
  Product4/1 -> Add/3
  Product2/1 -> Add/2
  Product3/1 -> Add/1
  Demux/3 -> Product4/2
  Demux/2 -> Product3/2
  Demux/1 -> Product2/2
  Product1/1 -> Product2/1
  Product/1 -> Product3/1, Product1/1
  tau/1 -> Product4/1, Product1/2, Product/2, Product/1

== system test_WaveletTraj/TrajGen1/Compute Join Output/CalcRho ==
  tau : Inport
  tau1 : Inport  Port=2
  Constant : Constant  OutDataTypeStr=fixdt(1,w,f)
  Divide : Product  Inputs=*/  OutDataTypeStr=fixdt(1,w,f)  RndMeth=Nearest  SaturateOnIntegerOverflow=on
  Product : Product  OutDataTypeStr=fixdt(1,w,f)  RndMeth=Nearest  SaturateOnIntegerOverflow=on
  Saturation1 : Saturate  UpperLimit=2^(w-f-1)  LowerLimit=2^-f  OutDataTypeStr=fixdt(1,w,f)  RndMeth=Nearest
  Sum1 : Sum  Inputs=|+-  OutDataTypeStr=fixdt(1,w,f)  RndMeth=Nearest  SaturateOnIntegerOverflow=on
  Sum2 : Sum  Inputs=-+|  OutDataTypeStr=fixdt(1,w,f)  RndMeth=Nearest  SaturateOnIntegerOverflow=on
  Rho1 : Outport
  Rho2 : Outport  Port=2
  wires:
  Sum2/1 -> Rho2/1
  Saturation1/1 -> Divide/2
  Product/1 -> Sum2/1, Rho1/1
  Sum1/1 -> Product/2, Product/1
  Constant/1 -> Sum2/2, Sum1/2
  Divide/1 -> Sum1/1
  tau1/1 -> Saturation1/1
  tau/1 -> Divide/1

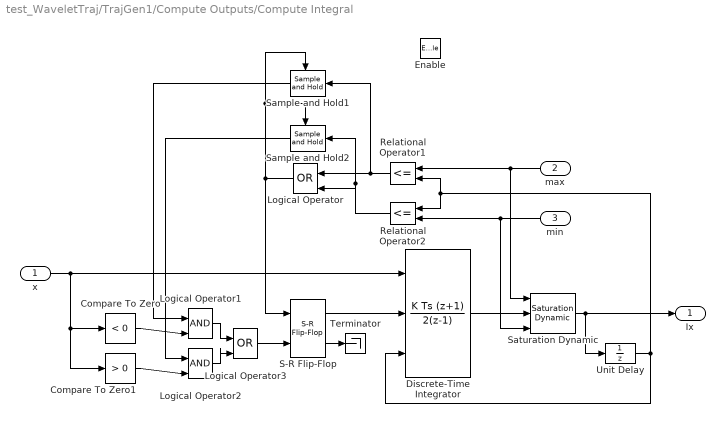
== system test_WaveletTraj/TrajGen1/Compute Outputs/Compute Integral ==
  x : Inport
  max : Inport  Port=2
  min : Inport  Port=3
  Enable : EnablePort
  Compare To Zero : simulink/Logic and Bit Operations/Compare To Zero  relop=<  OutDataTypeStr=boolean  ZeroCross=off
  Compare To Zero1 : simulink/Logic and Bit Operations/Compare To Zero  relop=>  OutDataTypeStr=boolean  ZeroCross=off
  Discrete-Time Integrator : DiscreteIntegrator  IntegratorMethod=Integration: Trapezoidal  ExternalReset=level  InitialConditionSource=external  SampleTime=Ts  OutDataTypeStr=fixdt(1,w,f)  RndMeth=Nearest  SaturateOnIntegerOverflow=on  ICPrevOutput=DiscIntNeverNeededParam  ICPrevScaledInput=DiscIntNeverNeededParam
  Logical Operator : Logic  Operator=OR  IconShape=distinctive  AllPortsSameDT=off  OutDataTypeStr=boolean
  Logical Operator1 : Logic  IconShape=distinctive  AllPortsSameDT=off  OutDataTypeStr=boolean
  Logical Operator2 : Logic  IconShape=distinctive  AllPortsSameDT=off  OutDataTypeStr=boolean
  Logical Operator3 : Logic  Operator=OR  IconShape=distinctive  AllPortsSameDT=off  OutDataTypeStr=boolean
  Relational Operator1 : RelationalOperator  Operator=<=  OutDataTypeStr=boolean  RndMeth=Nearest
  Relational Operator2 : RelationalOperator  Operator=<=  OutDataTypeStr=boolean  RndMeth=Nearest
  S-R Flip-Flop : simulink_extras/Flip Flops/S-R Flip-Flop  initial_condition=0
  Sample and Hold1 : dspsigops/Sample and Hold  trig=Either edge  initCond=0  latchinput=off
  Sample and Hold2 : dspsigops/Sample and Hold  trig=Either edge  initCond=0  latchinput=off
  Saturation Dynamic : simulink/Discontinuities/Saturation Dynamic  OutMin=[]  OutMax=[]  OutDataTypeStr=fixdt(1,w,f)  OutputDataTypeScalingMode=Specify via dialog  OutDataType=fixdt(1,w,f)  OutScaling=[]  RndMeth=Nearest  DoSatur=on
  Terminator : Terminator
  Unit Delay : UnitDelay  SampleTime=-1
  Ix : Outport
  wires:
  max/1 -> Relational Operator1/1, Saturation Dynamic/1
  min/1 -> Relational Operator2/2, Saturation Dynamic/3
  Relational Operator1/1 -> Logical Operator/1, Sample and Hold1/1
  Relational Operator2/1 -> Sample and Hold2/1, Logical Operator/2
  Discrete-Time Integrator/1 -> Saturation Dynamic/2
  Saturation Dynamic/1 -> Ix/1, Unit Delay/1
  x/1 -> Discrete-Time Integrator/1, Compare To Zero/1, Compare To Zero1/1
  Unit Delay/1 -> Discrete-Time Integrator/3, Relational Operator1/2, Relational Operator2/1
  S-R Flip-Flop/1 -> Discrete-Time Integrator/2
  S-R Flip-Flop/2 -> Terminator/1
  Logical Operator/1 -> S-R Flip-Flop/1, Sample and Hold1/Trigger, Sample and Hold2/Trigger
  Compare To Zero/1 -> Logical Operator1/2
  Compare To Zero1/1 -> Logical Operator2/2
  Logical Operator1/1 -> Logical Operator3/1
  Logical Operator2/1 -> Logical Operator3/2
  Logical Operator3/1 -> S-R Flip-Flop/2
  Sample and Hold1/1 -> Logical Operator1/1
  Sample and Hold2/1 -> Logical Operator2/1

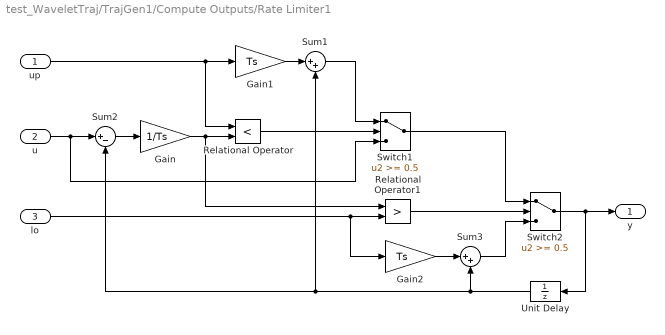
== system test_WaveletTraj/TrajGen1/Compute Outputs/Rate Limiter1 ==
  up : Inport
  u : Inport  Port=2
  lo : Inport  Port=3
  Gain : Gain  Gain=1/Ts  ParamDataTypeStr=fixdt(1,w,f)  RndMeth=Nearest  SaturateOnIntegerOverflow=on  OutDataTypeStr=Inherit: Same as input
  Gain1 : Gain  Gain=Ts  ParamDataTypeStr=fixdt(1,w,f)  OutDataTypeStr=fixdt(1,w,f)  RndMeth=Nearest  SaturateOnIntegerOverflow=on
  Gain2 : Gain  Gain=Ts  ParamDataTypeStr=fixdt(1,w,f)  OutDataTypeStr=fixdt(1,w,f)  RndMeth=Nearest  SaturateOnIntegerOverflow=on
  Relational Operator : RelationalOperator  Operator=<  OutDataTypeStr=boolean  RndMeth=Nearest
  Relational Operator1 : RelationalOperator  Operator=>  OutDataTypeStr=boolean  RndMeth=Nearest
  Sum1 : Sum  Inputs=|++  OutDataTypeStr=fixdt(1,w,f)  RndMeth=Nearest  SaturateOnIntegerOverflow=on
  Sum2 : Sum  Inputs=|+-  OutDataTypeStr=fixdt(1,w,f)  RndMeth=Nearest  SaturateOnIntegerOverflow=on
  Sum3 : Sum  Inputs=|++  OutDataTypeStr=fixdt(1,w,f)  RndMeth=Nearest  SaturateOnIntegerOverflow=on
  Switch1 : Switch  Threshold=0.5  OutDataTypeStr=fixdt(1,w,f)  RndMeth=Nearest  SaturateOnIntegerOverflow=on
  Switch2 : Switch  Threshold=0.5  OutDataTypeStr=fixdt(1,w,f)  RndMeth=Nearest  SaturateOnIntegerOverflow=on
  Unit Delay : UnitDelay  SampleTime=-1
  y : Outport
  wires:
  u/1 -> Sum2/1, Switch1/3
  Sum2/1 -> Gain/1
  Unit Delay/1 -> Sum2/2, Sum1/2, Sum3/2
  Gain/1 -> Relational Operator/2, Relational Operator1/1
  up/1 -> Relational Operator/1, Gain1/1
  Relational Operator/1 -> Switch1/2
  Gain1/1 -> Sum1/1
  Sum1/1 -> Switch1/1
  Switch1/1 -> Switch2/1
  Switch2/1 -> y/1, Unit Delay/1
  Relational Operator1/1 -> Switch2/2
  lo/1 -> Relational Operator1/2, Gain2/1
  Gain2/1 -> Sum3/1
  Sum3/1 -> Switch2/3

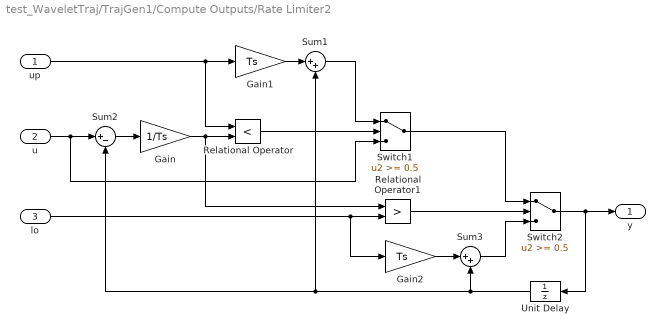
== system test_WaveletTraj/TrajGen1/Compute Outputs/Rate Limiter2 ==
  up : Inport
  u : Inport  Port=2
  lo : Inport  Port=3
  Gain : Gain  Gain=1/Ts  ParamDataTypeStr=fixdt(1,w,f)  RndMeth=Nearest  SaturateOnIntegerOverflow=on  OutDataTypeStr=Inherit: Same as input
  Gain1 : Gain  Gain=Ts  ParamDataTypeStr=fixdt(1,w,f)  OutDataTypeStr=fixdt(1,w,f)  RndMeth=Nearest  SaturateOnIntegerOverflow=on
  Gain2 : Gain  Gain=Ts  ParamDataTypeStr=fixdt(1,w,f)  OutDataTypeStr=fixdt(1,w,f)  RndMeth=Nearest  SaturateOnIntegerOverflow=on
  Relational Operator : RelationalOperator  Operator=<  OutDataTypeStr=boolean  RndMeth=Nearest
  Relational Operator1 : RelationalOperator  Operator=>  OutDataTypeStr=boolean  RndMeth=Nearest
  Sum1 : Sum  Inputs=|++  OutDataTypeStr=fixdt(1,w,f)  RndMeth=Nearest  SaturateOnIntegerOverflow=on
  Sum2 : Sum  Inputs=|+-  OutDataTypeStr=fixdt(1,w,f)  RndMeth=Nearest  SaturateOnIntegerOverflow=on
  Sum3 : Sum  Inputs=|++  OutDataTypeStr=fixdt(1,w,f)  RndMeth=Nearest  SaturateOnIntegerOverflow=on
  Switch1 : Switch  Threshold=0.5  OutDataTypeStr=fixdt(1,w,f)  RndMeth=Nearest  SaturateOnIntegerOverflow=on
  Switch2 : Switch  Threshold=0.5  OutDataTypeStr=fixdt(1,w,f)  RndMeth=Nearest  SaturateOnIntegerOverflow=on
  Unit Delay : UnitDelay  SampleTime=-1
  y : Outport
  wires:
  Sum3/1 -> Switch2/3
  Gain2/1 -> Sum3/1
  lo/1 -> Gain2/1, Relational Operator1/2
  Relational Operator1/1 -> Switch2/2
  Switch2/1 -> Unit Delay/1, y/1
  Switch1/1 -> Switch2/1
  Sum1/1 -> Switch1/1
  Gain1/1 -> Sum1/1
  Relational Operator/1 -> Switch1/2
  up/1 -> Gain1/1, Relational Operator/1
  Gain/1 -> Relational Operator1/1, Relational Operator/2
  Unit Delay/1 -> Sum3/2, Sum1/2, Sum2/2
  Sum2/1 -> Gain/1
  u/1 -> Switch1/3, Sum2/1

== system test_WaveletTraj/TrajGen1/Compute Position/Position ==
  Res : Inport
  tau : Inport  Port=2
  c : Inport  Port=3
  N : Inport  Port=4
  Position : Subsystem  RTWFcnName=Trajectory_Position
  out : Outport
  wires:
  N/1 -> Position/4(N)
  c/1 -> Position/3(c)
  Position/1(out) -> out/1
  tau/1 -> Position/2(tau)
  Res/1 -> Position/1(Res)

== system test_WaveletTraj/TrajGen1/Input Latching/Sample and Hold ==
  mode : Inport
  In : Inport  Port=2
  Trigger : TriggerPort  VariantControl=(inherit)  ZeroCross=off
  Constant : Constant  Value=2^3  OutDataTypeStr=fixdt(0,w,f)
  Constant1 : Constant  Value=2^4  OutDataTypeStr=fixdt(0,w,f)
  Data Type Conversion : DataTypeConversion  OutDataTypeStr=uint16  RndMeth=Ceiling  SaturateOnIntegerOverflow=on
  Multiport Switch : MultiPortSwitch  DataPortOrder=Zero-based contiguous  zeroidx=on  OutDataTypeStr=fixdt(0,w,f)  RndMeth=Nearest  SaturateOnIntegerOverflow=on
  " " : Outport  InitialOutput=initCond
  " 1" : Outport  Port=2  InitialOutput=initCond
  wires:
  Data Type Conversion/1 -> " 1"/1
  Multiport Switch/1 -> " "/1, Data Type Conversion/1
  mode/1 -> Multiport Switch/1
  In/1 -> Multiport Switch/2
  Constant/1 -> Multiport Switch/3
  Constant1/1 -> Multiport Switch/4

== system test_WaveletTraj/TrajGen1/Input Latching/Sample and Hold2 ==
  In : Inport
  Trigger : TriggerPort  VariantControl=(inherit)  ZeroCross=off
  Data Type Conversion : DataTypeConversion  OutDataTypeStr=uint32  SaturateOnIntegerOverflow=on
  Gain : Gain  Gain=1/Ts  ParamDataTypeStr=fixdt(1,w,f)  OutDataTypeStr=fixdt(1,w,f)  RndMeth=Nearest  SaturateOnIntegerOverflow=on
  " " : Outport  InitialOutput=initCond
  wires:
  Data Type Conversion/1 -> " "/1
  Gain/1 -> Data Type Conversion/1
  In/1 -> Gain/1

== system test_WaveletTraj/TrajGen1/Input Latching/Sample and Hold4 ==
  mode : Inport
  In : Inport  Port=2
  Trigger : TriggerPort  VariantControl=(inherit)  ZeroCross=off
  Multiport Switch : MultiPortSwitch  DataPortOrder=Zero-based contiguous  zeroidx=on  OutDataTypeStr=fixdt(1,w,f)  RndMeth=Nearest  SaturateOnIntegerOverflow=on
  constant : Constant  Value="[0.0156906989743308,  0.104549075132343,  0.277142440037961,  0.502199121925297,  0.726584938978675,  0.897421193763573,  0.982811374526835,  0.999579465917557,  1.00001660256494,  zeros(1,c_maxsz-9)]"  OutDataTypeStr=fixdt(1,w,f)
  constant1 : Constant  Value="[0.704980465851185,  0.994792363880808,  1.00001660256494*ones(1,15),  zeros(1,c_maxsz-17)]"  OutDataTypeStr=fixdt(1,w,f)
  " " : Outport  InitialOutput=initCond
  wires:
  Multiport Switch/1 -> " "/1
  mode/1 -> Multiport Switch/1
  In/1 -> Multiport Switch/2
  constant/1 -> Multiport Switch/3
  constant1/1 -> Multiport Switch/4

== system test_WaveletTraj/TrajGen1/Input Latching/Sample and Hold5 ==
  mode : Inport
  x0 : Inport  Port=2
  xf : Inport  Port=3
  Trigger : TriggerPort  VariantControl=(inherit)  ZeroCross=off
  Constant : Constant  OutDataTypeStr=fixdt(1,w,f)
  Sum2 : Sum  Inputs=-+|  OutDataTypeStr=fixdt(1,w,f)  RndMeth=Nearest  SaturateOnIntegerOverflow=on
  Switch1 : Switch  Threshold=0.5  OutDataTypeStr=fixdt(1,w,f)  RndMeth=Nearest  SaturateOnIntegerOverflow=on
  " " : Outport  InitialOutput=initCond
  wires:
  x0/1 -> Sum2/1
  xf/1 -> Sum2/2
  mode/1 -> Switch1/2
  Sum2/1 -> Switch1/1
  Switch1/1 -> " "/1
  Constant/1 -> Switch1/3

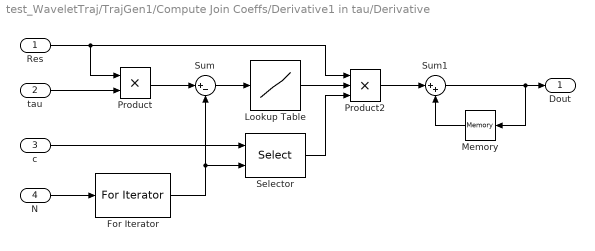
== system test_WaveletTraj/TrajGen1/Compute Join Coeffs/Derivative1 in tau/Derivative ==
  Res : Inport  PortDimensions=1
  tau : Inport  Port=2  PortDimensions=1
  c : Inport  Port=3  PortDimensions=c_maxsz
  N : Inport  Port=4  PortDimensions=1
  For Iterator : ForIterator  ResetStates=reset  IterationSource=external  IndexMode=Zero-based  IterationVariableDataType=int8
  Lookup Table : Lookup  InputValues=tval_fi  Table=Dphival_fi  LookUpMeth=Interpolation-Use End Values  RndMeth=Nearest  SaturateOnIntegerOverflow=on
  Memory : Memory  InheritSampleTime=on
  Product : Product  OutDataTypeStr=fixdt(1,w,f)  RndMeth=Nearest  SaturateOnIntegerOverflow=on
  Product2 : Product  Inputs=3  OutDataTypeStr=fixdt(1,w,f)  RndMeth=Nearest  SaturateOnIntegerOverflow=on
  Selector : Selector  IndexMode=Zero-based  InputPortWidth=c_maxsz  IndexOptions=Index vector (port)  Indices=[1 3]  OutputSizes=1
  Sum : Sum  Inputs=|+-  OutDataTypeStr=fixdt(1,w,f)  RndMeth=Nearest  SaturateOnIntegerOverflow=on
  Sum1 : Sum  Inputs=|++  OutDataTypeStr=fixdt(1,w,f)  RndMeth=Nearest  SaturateOnIntegerOverflow=on
  Dout : Outport  PortDimensions=1  InitialOutput=0
  wires:
  Product2/1 -> Sum1/1
  Selector/1 -> Product2/3
  Lookup Table/1 -> Product2/2
  Sum1/1 -> Memory/1, Dout/1
  Memory/1 -> Sum1/2
  c/1 -> Selector/1
  For Iterator/1 -> Selector/2, Sum/2
  N/1 -> For Iterator/1
  Product/1 -> Sum/1
  Sum/1 -> Lookup Table/1
  Res/1 -> Product2/1, Product/1
  tau/1 -> Product/2

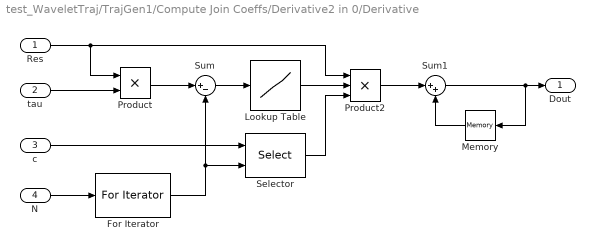
== system test_WaveletTraj/TrajGen1/Compute Join Coeffs/Derivative2 in 0/Derivative ==
  Res : Inport  PortDimensions=1
  tau : Inport  Port=2  PortDimensions=1
  c : Inport  Port=3  PortDimensions=c_maxsz
  N : Inport  Port=4  PortDimensions=1
  For Iterator : ForIterator  ResetStates=reset  IterationSource=external  IndexMode=Zero-based  IterationVariableDataType=int8
  Lookup Table : Lookup  InputValues=tval_fi  Table=Dphival_fi  LookUpMeth=Interpolation-Use End Values  RndMeth=Nearest  SaturateOnIntegerOverflow=on
  Memory : Memory  InheritSampleTime=on
  Product : Product  OutDataTypeStr=fixdt(1,w,f)  RndMeth=Nearest  SaturateOnIntegerOverflow=on
  Product2 : Product  Inputs=3  OutDataTypeStr=fixdt(1,w,f)  RndMeth=Nearest  SaturateOnIntegerOverflow=on
  Selector : Selector  IndexMode=Zero-based  InputPortWidth=c_maxsz  IndexOptions=Index vector (port)  Indices=[1 3]  OutputSizes=1
  Sum : Sum  Inputs=|+-  OutDataTypeStr=fixdt(1,w,f)  RndMeth=Nearest  SaturateOnIntegerOverflow=on
  Sum1 : Sum  Inputs=|++  OutDataTypeStr=fixdt(1,w,f)  RndMeth=Nearest  SaturateOnIntegerOverflow=on
  Dout : Outport  PortDimensions=1  InitialOutput=0
  wires:
  tau/1 -> Product/2
  Res/1 -> Product/1, Product2/1
  Sum/1 -> Lookup Table/1
  Product/1 -> Sum/1
  N/1 -> For Iterator/1
  For Iterator/1 -> Sum/2, Selector/2
  c/1 -> Selector/1
  Memory/1 -> Sum1/2
  Sum1/1 -> Dout/1, Memory/1
  Lookup Table/1 -> Product2/2
  Selector/1 -> Product2/3
  Product2/1 -> Sum1/1

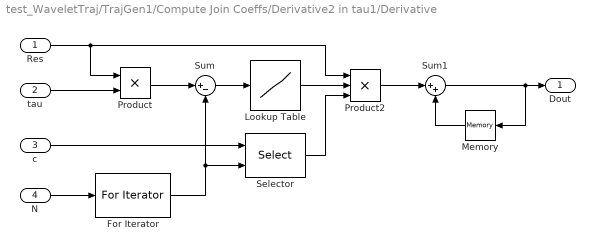
== system test_WaveletTraj/TrajGen1/Compute Join Coeffs/Derivative2 in tau1/Derivative ==
  Res : Inport  PortDimensions=1
  tau : Inport  Port=2  PortDimensions=1
  c : Inport  Port=3  PortDimensions=c_maxsz
  N : Inport  Port=4  PortDimensions=1
  For Iterator : ForIterator  ResetStates=reset  IterationSource=external  IndexMode=Zero-based  IterationVariableDataType=int8
  Lookup Table : Lookup  InputValues=tval_fi  Table=Dphival_fi  LookUpMeth=Interpolation-Use End Values  RndMeth=Nearest  SaturateOnIntegerOverflow=on
  Memory : Memory  InheritSampleTime=on
  Product : Product  OutDataTypeStr=fixdt(1,w,f)  RndMeth=Nearest  SaturateOnIntegerOverflow=on
  Product2 : Product  Inputs=3  OutDataTypeStr=fixdt(1,w,f)  RndMeth=Nearest  SaturateOnIntegerOverflow=on
  Selector : Selector  IndexMode=Zero-based  InputPortWidth=c_maxsz  IndexOptions=Index vector (port)  Indices=[1 3]  OutputSizes=1
  Sum : Sum  Inputs=|+-  OutDataTypeStr=fixdt(1,w,f)  RndMeth=Nearest  SaturateOnIntegerOverflow=on
  Sum1 : Sum  Inputs=|++  OutDataTypeStr=fixdt(1,w,f)  RndMeth=Nearest  SaturateOnIntegerOverflow=on
  Dout : Outport  PortDimensions=1  InitialOutput=0
  wires:
  Product2/1 -> Sum1/1
  Selector/1 -> Product2/3
  Lookup Table/1 -> Product2/2
  Sum1/1 -> Memory/1, Dout/1
  Memory/1 -> Sum1/2
  c/1 -> Selector/1
  For Iterator/1 -> Selector/2, Sum/2
  N/1 -> For Iterator/1
  Product/1 -> Sum/1
  Sum/1 -> Lookup Table/1
  Res/1 -> Product2/1, Product/1
  tau/1 -> Product/2

== system test_WaveletTraj/TrajGen1/Compute Join Coeffs/Position2 in tau1/Position ==
  Res : Inport  PortDimensions=1
  tau : Inport  Port=2  PortDimensions=1
  c : Inport  Port=3  PortDimensions=c_maxsz
  N : Inport  Port=4  PortDimensions=1
  For Iterator : ForIterator  ResetStates=reset  IterationSource=external  IndexMode=Zero-based  IterationVariableDataType=int8
  Lookup Table : Lookup  InputValues=tval_fi  Table=phival_fi  LookUpMeth=Interpolation-Use End Values  RndMeth=Nearest  SaturateOnIntegerOverflow=on
  Memory : Memory  InheritSampleTime=on
  Product : Product  OutDataTypeStr=fixdt(1,w,f)  RndMeth=Nearest  SaturateOnIntegerOverflow=on
  Product1 : Product  OutDataTypeStr=fixdt(1,w,f)  RndMeth=Nearest  SaturateOnIntegerOverflow=on
  Selector : Selector  IndexMode=Zero-based  InputPortWidth=c_maxsz  IndexOptions=Index vector (port)  Indices=[1 3]  OutputSizes=1
  Sum : Sum  Inputs=|+-  OutDataTypeStr=fixdt(1,w,f)  RndMeth=Nearest  SaturateOnIntegerOverflow=on
  Sum1 : Sum  Inputs=|++  OutDataTypeStr=fixdt(1,w,f)  RndMeth=Nearest  SaturateOnIntegerOverflow=on
  out : Outport  PortDimensions=1  InitialOutput=0
  wires:
  tau/1 -> Product/2
  Res/1 -> Product/1
  Sum/1 -> Lookup Table/1
  Product/1 -> Sum/1
  N/1 -> For Iterator/1
  For Iterator/1 -> Sum/2, Selector/2
  Lookup Table/1 -> Product1/1
  c/1 -> Selector/1
  Selector/1 -> Product1/2
  Product1/1 -> Sum1/1
  Memory/1 -> Sum1/2
  Sum1/1 -> out/1, Memory/1

== system test_WaveletTraj/TrajGen1/Compute Position/Position/Position ==
  Res : Inport  PortDimensions=1
  tau : Inport  Port=2  PortDimensions=1
  c : Inport  Port=3  PortDimensions=c_maxsz
  N : Inport  Port=4  PortDimensions=1
  For Iterator : ForIterator  ResetStates=reset  IterationSource=external  IndexMode=Zero-based  IterationVariableDataType=int8
  Lookup Table : Lookup  InputValues=tval_fi  Table=phival_fi  LookUpMeth=Interpolation-Use End Values  RndMeth=Nearest  SaturateOnIntegerOverflow=on
  Memory : Memory  InheritSampleTime=on
  Product : Product  OutDataTypeStr=fixdt(1,w,f)  RndMeth=Nearest  SaturateOnIntegerOverflow=on
  Product1 : Product  OutDataTypeStr=fixdt(1,w,f)  RndMeth=Nearest  SaturateOnIntegerOverflow=on
  Selector : Selector  IndexMode=Zero-based  InputPortWidth=c_maxsz  IndexOptions=Index vector (port)  Indices=[1 3]  OutputSizes=1
  Sum : Sum  Inputs=|+-  OutDataTypeStr=fixdt(1,w,f)  RndMeth=Nearest  SaturateOnIntegerOverflow=on
  Sum1 : Sum  Inputs=|++  OutDataTypeStr=fixdt(1,w,f)  RndMeth=Nearest  SaturateOnIntegerOverflow=on
  out : Outport  PortDimensions=1  InitialOutput=0
  wires:
  Sum1/1 -> Memory/1, out/1
  Memory/1 -> Sum1/2
  Product1/1 -> Sum1/1
  Selector/1 -> Product1/2
  c/1 -> Selector/1
  Lookup Table/1 -> Product1/1
  For Iterator/1 -> Selector/2, Sum/2
  N/1 -> For Iterator/1
  Product/1 -> Sum/1
  Sum/1 -> Lookup Table/1
  Res/1 -> Product/1
  tau/1 -> Product/2
